simulink model "vision"  (Simulink 9.1)
settings: Solver=ode45  StartTime=0.0  StopTime=10.0  RelTol=1e-3  EnableMultiTasking=on
undefined symbols (not defined in the file): none, Rec, SDTV, videoinput
libraries: visionanalysis x4, visiongeotforms x3, visionstatistics x1, visionconversions x1, visiontextngfix x1, imaqlib x1, dspindex x1
settings Model: SuppressorTable=22 serialization::archive 11 0 6 0 0 0 1 0  Creator=huber  LastModifiedBy=askar
settings DataIOCC: LimitDataPoints=on  SignalLoggingSaveFormat=ModelDataLogs
settings OptimizationCC: ExpressionDepthLimit=2147483647
settings DebuggingCC: SolverPrmCheckMsg=warning  FcnCallInpInsideContextMsg=warning  StateNameClashWarn=warning
settings GRTTargetCC: GeneratePreprocessorConditionals=Disable all  CombineOutputUpdateFcns=on  GRTInterface=off

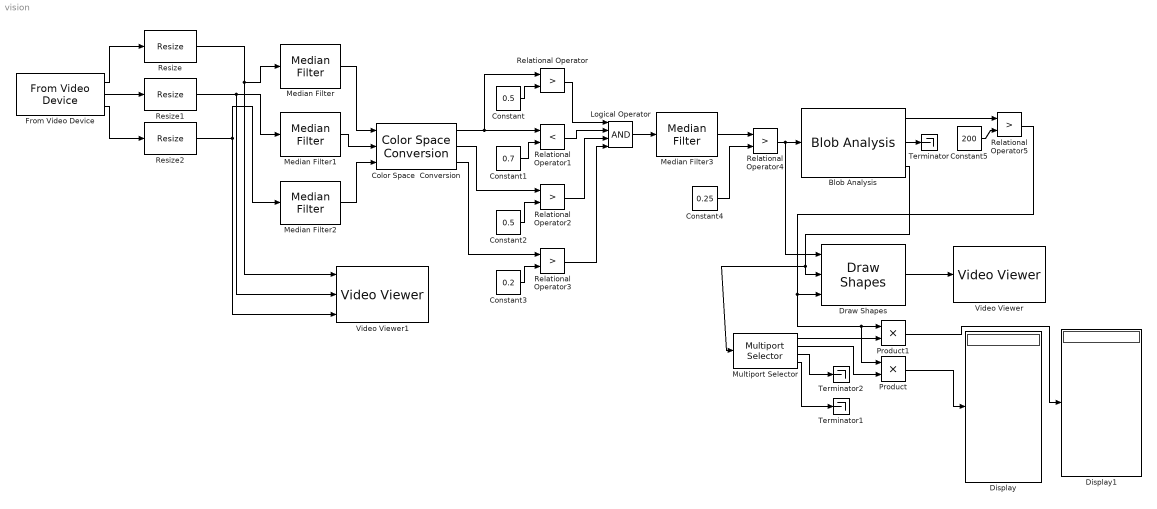
== system vision ==
  Blob Analysis : visionstatistics/Blob Analysis  Tag=vipblks_row_conv  area=on  centroid=on  bBox=on  majorAxis=off  minorAxis=off  angle=off  eccentricity=off  equivDiameterSq=off  extent=off  perimeter=off  maxBlobs=50  warnIfNumBlobsExceeded=on  isCount=off  useMinArea=off  minArea=0  useMaxArea=off  maxArea=intmax('uint32')  excludeBorderBlob=off  outDT=double  isOutVarDim=off  isFill=on  fillValues=-1  conn=8  isLabel=off  outputMode=Binary point scaling  outputWordLength=32  outputFracLength=16  firstCoeffMode=Binary point scaling  firstCoeffWordLength=16  firstCoeffFracLength=14  secondCoeffMode=Binary point scaling  secondCoeffWordLength=32  secondCoeffFracLength=16  accumMode=Binary point scaling  accumWordLength=32  accumFracLength=0  prodOutputMode=Binary point scaling  prodOutputWordLength=32  prodOutputFracLength=16  roundingMode=Floor  overflowMode=off
      settings: SourceProductName=Computer Vision System Toolbox
  Color Space  Conversion : visionconversions/Color Space  Conversion  conversion=Obsolete  conversionActive=R'G'B' to HSV  wp_str=D65  rec=Rec. 601 (SDTV)  sys=1125/60/2:1  imagePorts=Separate color signals
      settings: SourceProductName=Computer Vision System Toolbox
  Constant : Constant  Value=0.5
  Constant1 : Constant  Value=0.7
  Constant2 : Constant  Value=0.5
  Constant3 : Constant  Value=0.2
  Constant4 : Constant  Value=0.25
  Constant5 : Constant  Value=200
  Display : Display
  Display1 : Display
  Draw Shapes : visiontextngfix/Draw Shapes  shape=Rectangles  fill=off  lineWidth=1  fillClrSource=Input port  display=User-specified value  intensity=200  color=255  opacity=0.6  viewport=Entire image  antialiasing=off  inType=Obsolete  imagePorts=One multidimensional signal  prodOutputMode=Binary point scaling  prodOutputWordLength=32  prodOutputFracLength=14  memoryMode=Specify word length  memoryWordLength=16  memoryFracLength=15  roundingMode=Floor  overflowMode=off
      settings: SourceProductName=Computer Vision System Toolbox
  From Video Device : imaqlib/From Video Device  DeviceMenu=linuxvideo 1 (HD Pro Webcam C920)  Device=linuxvideo 1 (HD Pro Webcam C920)  ObjConstructor=videoinput('linuxvideo', 1)  VideoFormatMenu=RGB24_1280x720  VideoFormat=RGB24_1280x720  VideoSource=Source  ROIPosition=[0 0 720 1280]  EnableHWTrigger=off  TriggerConfiguration=none/none  SampleTime=1/10  OutputPortsMode=Separate color signals  DataType=single  CanDoHWTrigger=no  ReturnedColorSpace=rgb  BlockHandle=15.0011  ROIWidth=1280  ROIHeight=720  ROIColumn=0  ROIRow=0  EngXMLPath=/usr/local/MATLAB/R2018a/toolbox/imaq/imaq/private  DevXMLPath=/home/askar/Documents/MATLAB/SupportPackages/R2018a/toolbox/imaq/supportpackages/genericvideo/adaptor/glnxa64  EngLibPath=/usr/local/MATLAB/R2018a/toolbox/imaq/imaqblks/imaqmex/glnxa64  ColorSpace=rgb  BayerSensorAlignment=grbg
      settings: SourceProductName=Image Acquisition Toolbox
  Logical Operator : Logic  Inputs=4  AllPortsSameDT=off  OutDataTypeStr=boolean
  Median Filter : visionanalysis/Median Filter  nghbood=[5 5]  outSize=Same as input port I  padType=Constant  padSrc=Specify via dialog  padVal=0  roundingMode=Floor  overflowMode=off
      settings: SourceProductName=Computer Vision System Toolbox  SourceProductBaseCode=VP
  Median Filter1 : visionanalysis/Median Filter  nghbood=[5 5]  outSize=Same as input port I  padType=Constant  padSrc=Specify via dialog  padVal=0  roundingMode=Floor  overflowMode=off
      settings: SourceProductName=Computer Vision System Toolbox  SourceProductBaseCode=VP
  Median Filter2 : visionanalysis/Median Filter  nghbood=[5 5]  outSize=Same as input port I  padType=Constant  padSrc=Specify via dialog  padVal=0  roundingMode=Floor  overflowMode=off
      settings: SourceProductName=Computer Vision System Toolbox  SourceProductBaseCode=VP
  Median Filter3 : visionanalysis/Median Filter  nghbood=[7 7]  outSize=Same as input port I  padType=Constant  padSrc=Specify via dialog  padVal=0  roundingMode=Floor  overflowMode=off
      settings: SourceProductName=Computer Vision System Toolbox  SourceProductBaseCode=VP
  Multiport Selector : dspindex/Multiport Selector  rowsOrCols=Columns  idxCellArray={1 2 3 4}  idxErrMode=Clip Index
  Product : Product  RndMeth=Zero
  Product1 : Product  RndMeth=Zero
  Relational Operator{,2..5} (5 alike) : RelationalOperator  Operator=>  OutDataTypeStr=boolean  RndMeth=Nearest
  Relational Operator1 : RelationalOperator  Operator=<  OutDataTypeStr=boolean  RndMeth=Nearest
  Resize : visiongeotforms/Resize  specify=Number of output columns and preserve aspect ratio  rfactor=[200 150]  outCols=320  outRows=25  outRowsCols=[25 35]  interp_method=Nearest neighbor  antialias=off  useROI=off  roiFlag=off  prodOutputMode=Binary point scaling  prodOutputWordLength=32  prodOutputFracLength=10  roundingMode=Nearest  overflowMode=on
      settings: SourceProductName=Computer Vision System Toolbox  SourceProductBaseCode=VP
  Resize1 : visiongeotforms/Resize  specify=Number of output columns and preserve aspect ratio  rfactor=[200 150]  outCols=320  outRows=25  outRowsCols=[25 35]  interp_method=Nearest neighbor  antialias=off  useROI=off  roiFlag=off  prodOutputMode=Binary point scaling  prodOutputWordLength=32  prodOutputFracLength=10  roundingMode=Nearest  overflowMode=on
      settings: SourceProductName=Computer Vision System Toolbox  SourceProductBaseCode=VP
  Resize2 : visiongeotforms/Resize  specify=Number of output columns and preserve aspect ratio  rfactor=[200 150]  outCols=320  outRows=25  outRowsCols=[25 35]  interp_method=Nearest neighbor  antialias=off  useROI=off  roiFlag=off  prodOutputMode=Binary point scaling  prodOutputWordLength=32  prodOutputFracLength=10  roundingMode=Nearest  overflowMode=on
      settings: SourceProductName=Computer Vision System Toolbox  SourceProductBaseCode=VP
  Terminator : Terminator
  Terminator1 : Terminator
  Terminator2 : Terminator
  Video Viewer : VideoViewer  FigPos=[92 789 563 484]
  Video Viewer1 : VideoViewer  imagePorts=separate color signals  FigPos=[740 869 611 430]
  wires:
  From Video Device/1 -> Resize/1
  From Video Device/2 -> Resize1/1
  From Video Device/3 -> Resize2/1
  Median Filter/1 -> Color Space  Conversion/1
  Median Filter1/1 -> Color Space  Conversion/2
  Median Filter2/1 -> Color Space  Conversion/3
  Constant1/1 -> Relational Operator1/2
  Color Space  Conversion/1 -> Relational Operator/1, Relational Operator1/1
  Constant/1 -> Relational Operator/2
  Relational Operator/1 -> Logical Operator/1
  Logical Operator/1 -> Median Filter3/1
  Color Space  Conversion/2 -> Relational Operator2/1
  Constant2/1 -> Relational Operator2/2
  Color Space  Conversion/3 -> Relational Operator3/1
  Constant3/1 -> Relational Operator3/2
  Relational Operator1/1 -> Logical Operator/2
  Relational Operator2/1 -> Logical Operator/3
  Relational Operator3/1 -> Logical Operator/4
  Median Filter3/1 -> Relational Operator4/1
  Constant4/1 -> Relational Operator4/2
  Relational Operator4/1 -> Blob Analysis/1, Draw Shapes/1
  Draw Shapes/1 -> Video Viewer/1
  Constant5/1 -> Relational Operator5/2
  Blob Analysis/1 -> Relational Operator5/1
  Blob Analysis/3 -> Draw Shapes/2, Multiport Selector/1
  Relational Operator5/1 -> Draw Shapes/3, Product1/1, Product/1
  Blob Analysis/2 -> Terminator/1
  Multiport Selector/3 -> Terminator2/1
  Multiport Selector/4 -> Terminator1/1
  Multiport Selector/2 -> Product/2
  Product/1 -> Display/1
  Multiport Selector/1 -> Product1/2
  Product1/1 -> Display1/1
  Resize/1 -> Median Filter/1, Video Viewer1/1
  Resize1/1 -> Video Viewer1/2, Median Filter1/1
  Resize2/1 -> Median Filter2/1, Video Viewer1/3
